simulink model "sys_sp2_clp"  (Simulink 7.2)
settings: Solver=ode3  StartTime=0.0  StopTime=15  FixedStep=mws_designpoint.Timestep  RelTol=1e-3
values from neighbouring files (symbols this model uses):
  fc = 1/2*0    (= 0)    [my_ex1.m]
  Kb = 4    [my_ex1.m]
  sys_sp2 = ss(Alon_sp2,Blon_sp2,eye(2),[0 0]')    [my_ex2.m]
undefined symbols (not defined in the file or in its folder): K
libraries: aeroutilslib x1
settings Model: Creator=E183308  LastModifiedBy=E183308
settings DataIOCC: LimitDataPoints=off

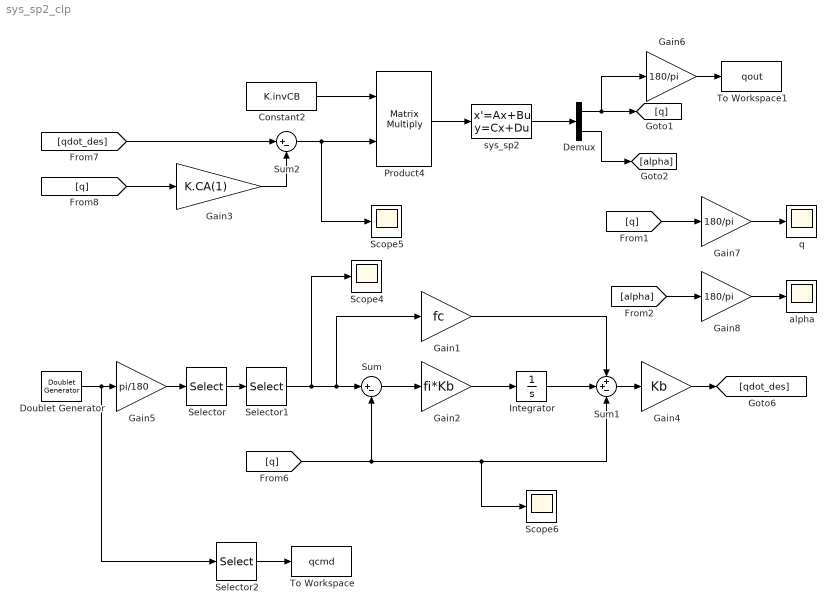
== system sys_sp2_clp ==
  Constant2 : Constant  Value=K.invCB  OutDataType=sfix(16)  OutScaling=2^0
  Demux : Demux  Outputs=2
  Doublet Generator : aeroutilslib/Doublet Generator  SystemSampleTime=-1  timeon=[2 0 0]  pulsewidth=[4 0 0]  amplitude=[0.500000 0.000000 0.000000]
  Gain1 : Gain  Gain=fc  ParameterDataType=sfix(16)  ParameterScaling=2^0  OutDataType=sfix(16)  OutScaling=2^0  SaturateOnIntegerOverflow=on  OutDataTypeStr=Inherit: Same as input  ParamDataTypeStr=Inherit: Same as input
  Gain2 : Gain  Gain=fi*Kb  ParameterDataType=sfix(16)  ParameterScaling=2^0  OutDataType=sfix(16)  OutScaling=2^0  SaturateOnIntegerOverflow=on  OutDataTypeStr=Inherit: Same as input  ParamDataTypeStr=Inherit: Same as input
  Gain3 : Gain  Gain=K.CA(1)  ParameterDataType=sfix(16)  ParameterScaling=2^0  OutDataType=sfix(16)  OutScaling=2^0  SaturateOnIntegerOverflow=on  OutDataTypeStr=Inherit: Same as input  ParamDataTypeStr=Inherit: Same as input
  Gain4 : Gain  Gain=Kb  ParameterDataType=sfix(16)  ParameterScaling=2^0  OutDataType=sfix(16)  OutScaling=2^0  SaturateOnIntegerOverflow=on  OutDataTypeStr=Inherit: Same as input  ParamDataTypeStr=Inherit: Same as input
  Gain5 : Gain  Gain=pi/180  ParameterDataType=sfix(16)  ParameterScaling=2^0  OutDataType=sfix(16)  OutScaling=2^0  SaturateOnIntegerOverflow=on  OutDataTypeStr=Inherit: Same as input  ParamDataTypeStr=Inherit: Same as input
  Gain6 : Gain  Gain=180/pi  ParameterDataType=sfix(16)  ParameterScaling=2^0  OutDataType=sfix(16)  OutScaling=2^0  SaturateOnIntegerOverflow=on  OutDataTypeStr=Inherit: Same as input  ParamDataTypeStr=Inherit: Same as input
  Gain7 : Gain  Gain=180/pi  ParameterDataType=sfix(16)  ParameterScaling=2^0  OutDataType=sfix(16)  OutScaling=2^0  SaturateOnIntegerOverflow=on  OutDataTypeStr=Inherit: Same as input  ParamDataTypeStr=Inherit: Same as input
  Gain8 : Gain  Gain=180/pi  ParameterDataType=sfix(16)  ParameterScaling=2^0  OutDataType=sfix(16)  OutScaling=2^0  SaturateOnIntegerOverflow=on  OutDataTypeStr=Inherit: Same as input  ParamDataTypeStr=Inherit: Same as input
  Integrator : Integrator
  Product4 : Product  Multiplication=Matrix(*)  OutDataType=sfix(16)  OutScaling=2^0  RndMeth=Zero
  Scope4 : Scope
      settings: YMin=-0.01  YMax=0.01
  Scope5 : Scope
      settings: YMin=-0.05  YMax=0.08  SaveName=ScopeData2
  Scope6 : Scope
      settings: YMin=-0.008  YMax=0.007
  Selector : Selector  InputPortWidth=3  IndexOptions=Index vector (dialog)  Indices=[2 1 3]  OutputSizes=1
  Selector1 : Selector  InputPortWidth=3  IndexOptions=Index vector (dialog)  Indices=2  OutputSizes=1
  Selector2 : Selector  InputPortWidth=3  IndexOptions=Index vector (dialog)  Indices=1  OutputSizes=1
  Sum : Sum  Inputs=|+-  OutDataType=sfix(16)  OutScaling=2^0
  Sum1 : Sum  Inputs=++-  OutDataType=sfix(16)  OutScaling=2^0
  Sum2 : Sum  Inputs=|+-  OutDataType=sfix(16)  OutScaling=2^0
  To Workspace : ToWorkspace  VariableName=qcmd  SampleTime=-1  SaveFormat=Structure With Time
  To Workspace1 : ToWorkspace  VariableName=qout  SampleTime=-1  SaveFormat=Array
  alpha : Scope
      settings: YMin=-0.008  YMax=0.007  SaveName=ScopeData4
  q : Scope
      settings: YMin=-0.008  YMax=0.007  SaveName=ScopeData3
  sys_sp2 : StateSpace  A=sys_sp2.a  B=sys_sp2.b  C=sys_sp2.c  D=sys_sp2.d
  wires:
  Doublet Generator/1 -> Gain5/1, Selector2/1
  [q] -> Sum/2, Sum1/3, Scope6/1
  Sum/1 -> Gain2/1
  Gain2/1 -> Integrator/1
  Gain1/1 -> Sum1/1
  Integrator/1 -> Sum1/2
  Sum1/1 -> Gain4/1
  Gain4/1 -> [qdot_des]
  Gain5/1 -> Selector/1
  Selector/1 -> Selector1/1
  sys_sp2/1 -> Demux/1
  Demux/1 -> [q], Gain6/1
  Demux/2 -> [alpha]
  [qdot_des] -> Sum2/1
  Constant2/1 -> Product4/1
  Sum2/1 -> Product4/2, Scope5/1
  [q] -> Gain3/1
  Product4/1 -> sys_sp2/1
  Selector2/1 -> To Workspace/1
  Selector1/1 -> Sum/1, Gain1/1, Scope4/1
  Gain6/1 -> To Workspace1/1
  Gain3/1 -> Sum2/2
  Gain7/1 -> q/1
  Gain8/1 -> alpha/1
  [q] -> Gain7/1
  [alpha] -> Gain8/1
